simulink model "exam6"  (R2016a)
settings: Solver=VariableStepAuto  StartTime=0.0  StopTime=10.0  RelTol=1e-3
settings Model: Creator=linghao  LastModifiedBy=linghao
settings GRTTargetCC: GeneratePreprocessorConditionals=Use local settings

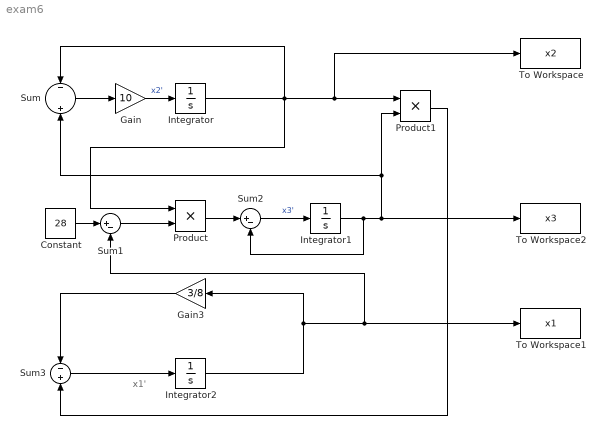
== system exam6 ==
  note: x1'
  Constant : Constant  Value=28
  Gain : Gain  Gain=10
  Gain3 : Gain  Gain=3/8
  Integrator : Integrator
  Integrator1 : Integrator
  Integrator2 : Integrator  InitialCondition=10^(-10)
  Product : Product
  Product1 : Product
  Sum : Sum  Inputs=-|||+
  Sum1 : Sum  Inputs=|+-
  Sum2 : Sum  Inputs=|+-
  Sum3 : Sum  Inputs=-+
  To Workspace : ToWorkspace  VariableName=x2  SampleTime=-1
  To Workspace1 : ToWorkspace  VariableName=x1  SampleTime=-1
  To Workspace2 : ToWorkspace  VariableName=x3  SampleTime=-1
  wires:
  Integrator/1 -> To Workspace/1, Product1/1, Product/1, Sum/1
  Sum/1 -> Gain/1
  Gain/1 -> Integrator/1  "x2'"
  Integrator1/1 -> Sum2/2, To Workspace2/1, Product1/2, Sum/2
  Integrator2/1 -> Gain3/1, To Workspace1/1, Sum1/2
  Sum1/1 -> Product/2
  Product/1 -> Sum2/1
  Sum2/1 -> Integrator1/1  "x3'"
  Sum3/1 -> Integrator2/1
  Gain3/1 -> Sum3/1
  Product1/1 -> Sum3/2
  Constant/1 -> Sum1/1
